simulink model "Integ_Model_Hepta"  (R2022a)
settings: configuration reference "VLS_Standard_Configuration" (kept outside this file)
undefined symbols (not defined in the file or in its folder): C_AFS_SpeedThrAct, C_AfsRampTimeMatrix, C_AnimationOnLoop, C_AnimationPeriod, C_AnimationPriority, C_CieCurveGammaToPwmY, C_CieCurvePwmToGammaY, C_CL_Ti_Speed_Hystresis, C_CL_Ti_Speed_Threshold, C_ClActAlgo, C_ClLeftSideTable_Alpha1, C_ClLeftSideTable_Alpha2, C_ClManeuverPwm, C_ClRightSideTable_Alpha1, C_ClRightSideTable_Alpha2, C_ClSpeedCurve, C_ClTableSize, C_ClTownPwm, C_Config, C_CSpeed0, C_DblDeadZone, C_DblEnable, C_DblInterDblAngValues, C_DblInterStwAngValues, C_DblLeftAngles, C_DblRampTime, C_DblRateLimit, C_DblRightAngles, C_DblSlavePeriod, C_DblSpeed0, C_DefaultValue, C_DrlRampTime, C_EndIndexOfEachLightingModule, C_EndValues, C_ForceExternalAfsMode, C_IndexOfStartStepForEachScenario, C_IsClOnTps, C_IsDblActive, C_IsDrlAutorizedInPower2, C_IsDrlPlOnTps, C_IsPlAutorizedInPower2, C_IsTiAutorizedInPower2, C_IsTiOnTps, C_LedCenterDist, C_LedCenterLimits, C_LedLeftDist, C_LedRightDist, C_LedStartIndexOfCl, C_LedStartIndexOfDrlPl, C_LedStartIndexOfTi, C_LeftDblMaxAngle, C_LeftDblMinAngle, C_MaintainAnimationPwm, C_MaintainAnimationTime, C_NumOfStepsForEachScenario, C_PlNominalPwm, C_PlOverDRL, C_RightDblMaxAngle, C_RightDblMinAngle, C_StartIndexOfEachLightingModule ... (+14)
libraries: simulink x11, AFS_MasterFeature x2, DodecaPreprocessingLib x1, Cl_Lib x1, DBL_MasterLib x1, AfsSlaveLib x1, DblSlaveLib x1, StdAnimationLibrary_R2020b x1, Ramp_Library_R2017b x1, STD_Signaling_Lib x1
(part 2 of 2)

== system Integ_Model_Hepta/Subsystem/Master/DBL_Master/Function-Call Subsystem ==
  V_FiltStWhAngleScaled : Inport
  V_DblEnable : Inport  Port=2
  V_FiltVehSpeed : Inport  Port=3
  function : TriggerPort  TriggerType=function-call  VariantControl=Variant
  Constant : Constant  Value=C_DblInterStwAngValues  VectorParams1D=off
  Constant1 : Constant  Value=C_DblDeadZone  VectorParams1D=off
  Constant2 : Constant  Value=C_DblInterDblAngValues  VectorParams1D=off
  Constant3 : Constant  Value=C_DblRateLimit  VectorParams1D=off
  Constant4 : Constant  Value=C_DblSpeed0  VectorParams1D=off
  Constant5 : Constant  Value=C_CSpeed0  VectorParams1D=off
  Constant6 : Constant  Value=C_LeftDblMinAngle  VectorParams1D=off
  Constant7 : Constant  Value=C_LeftDblMaxAngle  VectorParams1D=off
  Constant8 : Constant  Value=C_RightDblMinAngle  VectorParams1D=off
  Constant9 : Constant  Value=C_RightDblMaxAngle  VectorParams1D=off
  DblMasterLib : DBL_MasterLib/DblMasterLib  SystemSampleTime=-1  VariantActivationTime=update diagram  Latency=0  AutoFrameSizeCalculation=off
  V_LeftDblAimingAngle : Outport  VectorParamsAs1DForOutWhenUnconnected=off
  V_RightDblAimingAngle : Outport  Port=2  VectorParamsAs1DForOutWhenUnconnected=off
  wires:
  Constant7/1 -> DblMasterLib/11
  Constant4/1 -> DblMasterLib/8
  Constant6/1 -> DblMasterLib/10
  Constant9/1 -> DblMasterLib/13
  Constant5/1 -> DblMasterLib/9
  DblMasterLib/1 -> V_LeftDblAimingAngle/1
  V_DblEnable/1 -> DblMasterLib/2
  Constant2/1 -> DblMasterLib/4
  DblMasterLib/2 -> V_RightDblAimingAngle/1
  Constant1/1 -> DblMasterLib/5
  Constant/1 -> DblMasterLib/3
  V_FiltVehSpeed/1 -> DblMasterLib/7
  Constant3/1 -> DblMasterLib/6
  V_FiltStWhAngleScaled/1 -> DblMasterLib/1
  Constant8/1 -> DblMasterLib/12

== system Integ_Model_Hepta/Subsystem/SideDetection/SideDetectionManager/If Action Subsystem ==
  V_DblAimingAngleLeft : Inport
  V_CmdTiLeft : Inport  Port=2
  V_AfsMode : Inport  Port=3
  V_ClLeft : Inport  Port=4
  Action Port : ActionPort  ActionPortLabel=if(u1 == 0)
  V_DblAngle : Outport
  V_CmdTi : Outport  Port=2
  V_AfsLightingMode : Outport  Port=3
  V_ClActive : Outport  Port=4
  wires:
  V_DblAimingAngleLeft/1 -> V_DblAngle/1
  V_CmdTiLeft/1 -> V_CmdTi/1
  V_AfsMode/1 -> V_AfsLightingMode/1
  V_ClLeft/1 -> V_ClActive/1

== system Integ_Model_Hepta/Subsystem/SideDetection/SideDetectionManager/If Action Subsystem1 ==
  V_DblAimingAngleRight : Inport
  V_CmdTiRight : Inport  Port=2
  V_AfsModeCanIn : Inport  Port=3
  V_ClRight : Inport  Port=4
  Action Port : ActionPort  ActionPortLabel=else
  V_DblAngle : Outport
  V_CmdTi : Outport  Port=2
  V_AfsLightingMode : Outport  Port=3
  V_ClActive : Outport  Port=4
  wires:
  V_CmdTiRight/1 -> V_CmdTi/1
  V_DblAimingAngleRight/1 -> V_DblAngle/1
  V_AfsModeCanIn/1 -> V_AfsLightingMode/1
  V_ClRight/1 -> V_ClActive/1

== system Integ_Model_Hepta/Subsystem/Slave/AFS/ConvertAfsModetoSlave ==
  note: The requirement of different LB current
  V_ActiveLightingMode : Inport
  V_LowBeamRequest : Inport  Port=2
  Constant1 : Constant  Value=N_E_HBHighSpeed
  Constant12 : Constant  Value=N_E_HBLowSpeed
  Constant2 : Constant  Value=N_E_HBLowSpeed
  Constant21 : Constant  Value=0  OutDataTypeStr=Inherit: Inherit via back propagation
  Constant4 : Constant  Value=N_E_NoFunction
  Constant5 : Constant  Value=N_E_HBHighSpeed
  Constant6 : Constant  Value=0  OutDataTypeStr=Inherit: Inherit via back propagation
  Equal1 : RelationalOperator  Operator===  OutDataTypeStr=boolean  RndMeth=Simplest  InputSameDT=off
  Equal2 : RelationalOperator  Operator===  OutDataTypeStr=boolean  RndMeth=Simplest  InputSameDT=off
  Equal3 : RelationalOperator  Operator=~=  OutDataTypeStr=boolean  RndMeth=Simplest  InputSameDT=off
  Equal4 : RelationalOperator  Operator===  OutDataTypeStr=boolean  RndMeth=Simplest  InputSameDT=off
  Switch{,1..4} (5 alike) : Switch  Criteria=u2 ~= 0  SaturateOnIntegerOverflow=off  InputSameDT=off
  Vector Concatenate : Concatenate
  V_ActiveLightingModes : Outport
  wires:
  Switch/1 -> Vector Concatenate/2
  Constant12/1 -> Equal1/1, Switch3/1
  Constant21/1 -> Switch/1
  Vector Concatenate/1 -> V_ActiveLightingModes/1
  Equal2/1 -> Switch/2
  Switch1/1 -> Switch/3
  Equal3/1 -> Switch1/2
  Constant2/1 -> Switch2/1, Equal3/1
  V_ActiveLightingMode/1 -> Equal2/1, Equal3/2, Switch1/1, Equal1/2, Switch4/1, Equal4/1
  Switch2/1 -> Switch1/3
  V_LowBeamRequest/1 -> Switch2/2
  Constant4/1 -> Switch2/3
  Equal1/1 -> Switch3/2
  Switch3/1 -> Vector Concatenate/1
  Constant1/1 -> Equal2/2
  Switch4/1 -> Switch3/3
  Equal4/1 -> Switch4/2
  Constant5/1 -> Equal4/2
  Constant6/1 -> Switch4/3

== system Integ_Model_Hepta/Subsystem/Slave/Signaling/DrlPl ==
  Pl : Inport
  Drl : Inport  Port=2
  Constant : Constant  Value=C_PlNominalPwm
  Constant1 : Constant  Value=N_MaxPwm
  Constant2 : Constant  Value=0  OutDataTypeStr=Inherit: Inherit via back propagation
  Constant5 : Constant  Value=C_DrlRampTime
  Constant6 : Constant  Value=C_TeAdbSlave
  Constant7 : Constant  Value=C_CieCurvePwmToGammaY
  Constant8 : Constant  Value=C_CieCurveGammaToPwmY
  GammaRampLibraryPerLedGroup : Ramp_Library_R2017b/GammaRampLibraryPerLedGroup  Description=|  SystemSampleTime=-1  VariantActivationTime=update diagram  Latency=0  AutoFrameSizeCalculation=off
      | This library performs ramp function taking CIE curves which are evenly distributed.
      | It performs the ramp linearly on the Gamma Curve.
  Logical Operator : Logic  Operator=NOT  AllPortsSameDT=off  OutDataTypeStr=boolean
  Switch : Switch  Criteria=u2 ~= 0  OutDataTypeStr=Inherit: Inherit via back propagation  SaturateOnIntegerOverflow=off  InputSameDT=off
  Switch1 : Switch  Criteria=u2 ~= 0  OutDataTypeStr=Inherit: Inherit via back propagation  SaturateOnIntegerOverflow=off  InputSameDT=off
  Terminator : Terminator
  V_DrlPlTpsPwm : Outport
  wires:
  Switch/1 -> GammaRampLibraryPerLedGroup/1
  [Drl] -> Switch1/2
  Constant8/1 -> GammaRampLibraryPerLedGroup/6
  Constant1/1 -> Switch1/1
  Constant7/1 -> GammaRampLibraryPerLedGroup/5
  Drl/1 -> [Drl]
  Switch1/1 -> Switch/3
  Constant/1 -> Switch/1
  Constant5/1 -> GammaRampLibraryPerLedGroup/2
  [Drl] -> Logical Operator/1
  Constant6/1 -> GammaRampLibraryPerLedGroup/4
  Logical Operator/1 -> GammaRampLibraryPerLedGroup/3
  Constant2/1 -> Switch1/3
  Pl/1 -> Switch/2
  GammaRampLibraryPerLedGroup/2 -> Terminator/1
  GammaRampLibraryPerLedGroup/1 -> V_DrlPlTpsPwm/1

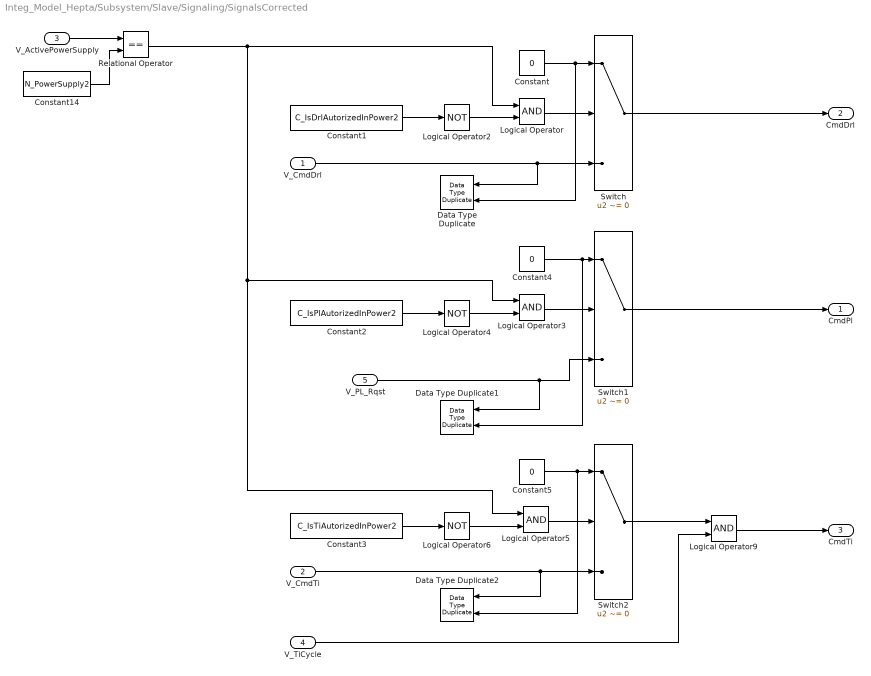
== system Integ_Model_Hepta/Subsystem/Slave/Signaling/SignalsCorrected ==
  "V_CmdDrl " : Inport
  V_CmdTi : Inport  Port=2
  V_ActivePowerSupply : Inport  Port=3
  V_TiCycle : Inport  Port=4
  V_PL_Rqst : Inport  Port=5
  Constant : Constant  Value=0  OutDataTypeStr=Inherit: Inherit via back propagation
  Constant1 : Constant  Value=C_IsDrlAutorizedInPower2
  Constant14 : Constant  Value=N_PowerSupply2
  Constant2 : Constant  Value=C_IsPlAutorizedInPower2
  Constant3 : Constant  Value=C_IsTiAutorizedInPower2
  Constant4 : Constant  Value=0  OutDataTypeStr=Inherit: Inherit via back propagation
  Constant5 : Constant  Value=0  OutDataTypeStr=Inherit: Inherit via back propagation
  Data Type Duplicate : DataTypeDuplicate
  Data Type Duplicate1 : DataTypeDuplicate
  Data Type Duplicate2 : DataTypeDuplicate
  Logical Operator{,3,5,9} (4 alike) : Logic  AllPortsSameDT=off  OutDataTypeStr=boolean
  Logical Operator2 : Logic  Operator=NOT  AllPortsSameDT=off  OutDataTypeStr=boolean
  Logical Operator4 : Logic  Operator=NOT  AllPortsSameDT=off  OutDataTypeStr=boolean
  Logical Operator6 : Logic  Operator=NOT  AllPortsSameDT=off  OutDataTypeStr=boolean
  Relational Operator : RelationalOperator  Operator===  OutDataTypeStr=boolean  RndMeth=Simplest  InputSameDT=off
  Switch : Switch  Criteria=u2 ~= 0  OutDataTypeStr=Inherit: Inherit via back propagation  SaturateOnIntegerOverflow=off  InputSameDT=off
  Switch1 : Switch  Criteria=u2 ~= 0  OutDataTypeStr=Inherit: Inherit via back propagation  SaturateOnIntegerOverflow=off  InputSameDT=off
  Switch2 : Switch  Criteria=u2 ~= 0  OutDataTypeStr=Inherit: Inherit via back propagation  SaturateOnIntegerOverflow=off  InputSameDT=off
  CmdPl : Outport
  CmdDrl : Outport  Port=2
  CmdTi : Outport  Port=3
  wires:
  Constant3/1 -> Logical Operator6/1
  V_TiCycle/1 -> Logical Operator9/2
  Switch1/1 -> CmdPl/1
  Switch2/1 -> Logical Operator9/1
  Logical Operator6/1 -> Logical Operator5/2
  Switch/1 -> CmdDrl/1
  Logical Operator9/1 -> CmdTi/1
  Logical Operator4/1 -> Logical Operator3/2
  V_ActivePowerSupply/1 -> Relational Operator/1
  Logical Operator3/1 -> Switch1/2
  Constant14/1 -> Relational Operator/2
  Relational Operator/1 -> Logical Operator5/1, Logical Operator3/1, Logical Operator/1
  Constant1/1 -> Logical Operator2/1
  "V_CmdDrl "/1 -> Data Type Duplicate/1, Switch/3
  Constant4/1 -> Data Type Duplicate1/2, Switch1/1
  Constant5/1 -> Data Type Duplicate2/2, Switch2/1
  V_PL_Rqst/1 -> Data Type Duplicate1/1, Switch1/3
  Logical Operator5/1 -> Switch2/2
  Logical Operator/1 -> Switch/2
  Logical Operator2/1 -> Logical Operator/2
  V_CmdTi/1 -> Data Type Duplicate2/1, Switch2/3
  Constant2/1 -> Logical Operator4/1
  Constant/1 -> Data Type Duplicate/2, Switch/1

== system Integ_Model_Hepta/Subsystem/Slave/Signaling/Ti ==
  Ti : Inport
  Constant3 : Constant  Value=N_MaxPwm
  Constant4 : Constant  Value=0  OutDataTypeStr=Inherit: Inherit via back propagation
  Switch2 : Switch  Criteria=u2 ~= 0  OutDataTypeStr=Inherit: Inherit via back propagation  SaturateOnIntegerOverflow=off  InputSameDT=off
  V_TiTpsPwm : Outport
  wires:
  Constant4/1 -> Switch2/3
  Constant3/1 -> Switch2/1
  Ti/1 -> Switch2/2
  Switch2/1 -> V_TiTpsPwm/1

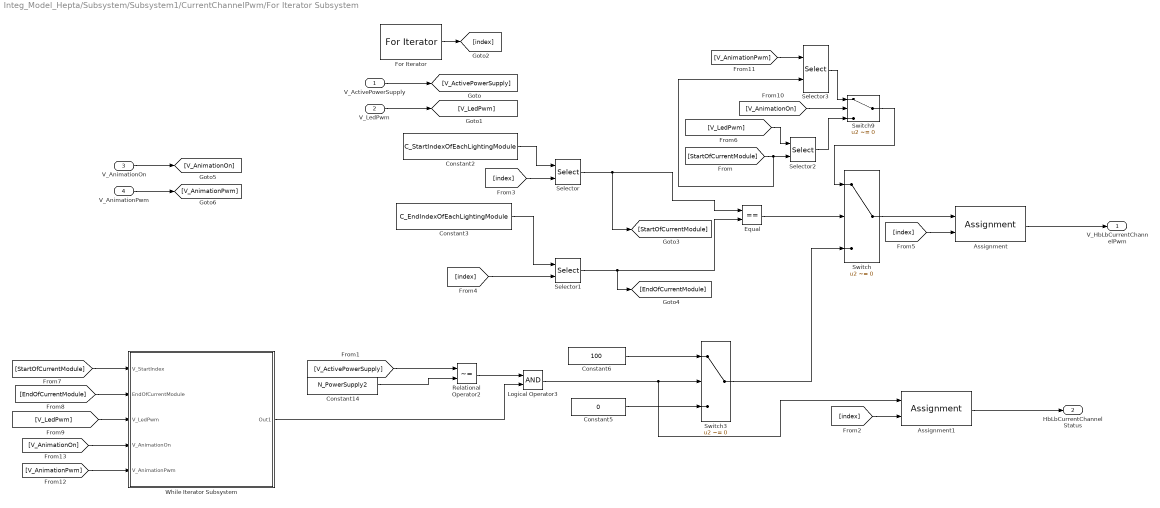
== system Integ_Model_Hepta/Subsystem/Subsystem1/CurrentChannelPwm/For Iterator Subsystem ==
  V_ActivePowerSupply : Inport
  V_LedPwm : Inport  Port=2
  V_AnimationOn : Inport  Port=3
  V_AnimationPwm : Inport  Port=4
  Assignment : Assignment  IndexMode=Zero-based  OutputInitialize=Specify size for each dimension in table  DiagnosticForDimensions=Error  IndexOptions=Starting index (port)  Indices=1  OutputSizes=C_NumOfLightingModules
  Assignment1 : Assignment  IndexMode=Zero-based  OutputInitialize=Specify size for each dimension in table  DiagnosticForDimensions=Error  IndexOptions=Starting index (port)  Indices=1  OutputSizes=C_NumOfLightingModules
  Constant14 : Constant  Value=N_PowerSupply2  OutDataTypeStr=Inherit: Inherit via back propagation
  Constant2 : Constant  Value=C_StartIndexOfEachLightingModule
  Constant3 : Constant  Value=C_EndIndexOfEachLightingModule
  Constant5 : Constant  Value=0
  Constant6 : Constant  Value=100  OutDataTypeStr=Inherit: Inherit via back propagation
  Equal : RelationalOperator  Operator===  OutDataTypeStr=boolean  RndMeth=Simplest  InputSameDT=off
  For Iterator : ForIterator  IterationLimit=C_NumOfLightingModules  IndexMode=Zero-based
  Logical Operator3 : Logic  AllPortsSameDT=off  OutDataTypeStr=boolean
  Relational Operator2 : RelationalOperator  Operator=~=  OutDataTypeStr=boolean  RndMeth=Simplest  InputSameDT=off
  Selector{,1..3} (4 alike) : Selector  IndexMode=Zero-based  IndexOptions=Index vector (port)  Indices=[1 3]  OutputSizes=1
  Switch : Switch  Criteria=u2 ~= 0  SaturateOnIntegerOverflow=off  InputSameDT=off
  Switch3 : Switch  Criteria=u2 ~= 0  SaturateOnIntegerOverflow=off  InputSameDT=off
  Switch9 : Switch  Criteria=u2 ~= 0  SaturateOnIntegerOverflow=off  InputSameDT=off
  While Iterator Subsystem : Subsystem  TreatAsAtomicUnit=on
  V_HbLbCurrentChannelPwm : Outport
  HbLbCurrentChannelStatus : Outport  Port=2
  wires:
  Selector/1 -> [StartOfCurrentModule], Equal/1
  Selector1/1 -> [EndOfCurrentModule], Equal/2
  Equal/1 -> Switch/2
  V_ActivePowerSupply/1 -> [V_ActivePowerSupply]
  V_LedPwm/1 -> [V_LedPwm]
  Selector2/1 -> Switch9/3
  Constant14/1 -> Relational Operator2/2
  Constant6/1 -> Switch3/1
  Switch3/1 -> Switch/3
  Relational Operator2/1 -> Logical Operator3/1
  Constant5/1 -> Switch3/3
  Logical Operator3/1 -> Assignment1/1, Switch3/2
  While Iterator Subsystem/1(Out1) -> Logical Operator3/2
  [V_ActivePowerSupply] -> Relational Operator2/1
  Switch/1 -> Assignment/1
  For Iterator/1 -> [index]
  [index] -> Selector/2
  [index] -> Selector1/2
  Constant2/1 -> Selector/1
  Constant3/1 -> Selector1/1
  Assignment/1 -> V_HbLbCurrentChannelPwm/1
  [index] -> Assignment/2
  [V_LedPwm] -> Selector2/1
  [StartOfCurrentModule] -> Selector3/2, Selector2/2
  [StartOfCurrentModule] -> While Iterator Subsystem/1(V_StartIndex)
  [EndOfCurrentModule] -> While Iterator Subsystem/2(EndOfCurrentModule)
  [V_LedPwm] -> While Iterator Subsystem/3(V_LedPwm)
  [index] -> Assignment1/2
  Assignment1/1 -> HbLbCurrentChannelStatus/1
  Selector3/1 -> Switch9/1
  V_AnimationPwm/1 -> [V_AnimationPwm]
  V_AnimationOn/1 -> [V_AnimationOn]
  [V_AnimationOn] -> Switch9/2
  [V_AnimationPwm] -> Selector3/1
  Switch9/1 -> Switch/1
  [V_AnimationPwm] -> While Iterator Subsystem/5(V_AnimationPwm)
  [V_AnimationOn] -> While Iterator Subsystem/4(V_AnimationOn)

== system Integ_Model_Hepta/Subsystem/Subsystem1/CurrentChannelPwm/Subsystem2 ==
  V_DrlPlFunctionTpsPwm : Inport
  V_PL_OUT : Inport  Port=2
  V_DRL_OUT : Inport  Port=3
  V_AnimationOn : Inport  Port=4
  If : If  NumInputs=2  IfExpression=u1==1  ElseIfExpressions=u2==1
  If Action Subsystem : Subsystem  TreatAsAtomicUnit=on
  If Action Subsystem1 : Subsystem  TreatAsAtomicUnit=on
  If Action Subsystem2 : Subsystem  TreatAsAtomicUnit=on
  IsNonZero : simulink/Logic and Bit Operations/Compare To Zero  relop=~=  OutDataTypeStr=boolean
  IsNonZero1 : simulink/Logic and Bit Operations/Compare To Zero  relop=~=  OutDataTypeStr=boolean
  Logical Operator : Logic  AllPortsSameDT=off  OutDataTypeStr=boolean
  Logical Operator1 : Logic  AllPortsSameDT=off  OutDataTypeStr=boolean
  Logical Operator2 : Logic  Operator=OR  AllPortsSameDT=off  OutDataTypeStr=boolean
  Merge : Merge  Inputs=3
  Channle_Status : Outport
  wires:
  V_PL_OUT/1 -> Logical Operator/2
  If/1 -> If Action Subsystem/Action
  Merge/1 -> Channle_Status/1
  V_DrlPlFunctionTpsPwm/1 -> Logical Operator/1, Logical Operator1/2
  If/2 -> If Action Subsystem1/Action
  Logical Operator1/1 -> IsNonZero1/1
  IsNonZero/1 -> If/2
  If/3 -> If Action Subsystem2/Action
  V_DRL_OUT/1 -> Logical Operator2/2
  If Action Subsystem2/1(Channle_Status) -> Merge/3
  Logical Operator/1 -> IsNonZero/1
  If Action Subsystem/1(Channle_Status) -> Merge/1
  IsNonZero1/1 -> If/1
  If Action Subsystem1/1(Channle_Status) -> Merge/2
  Logical Operator2/1 -> Logical Operator1/1
  V_AnimationOn/1 -> Logical Operator2/1

== system Integ_Model_Hepta/Subsystem/Master/AFS_Master/AFS_Master/AFS_Fail_safe_strategy ==
  V_CAN_Fail : Inport
  V_Veh_speed_Fail : Inport  Port=2
  V_Mod_LeftFail : Inport  Port=3
  V_Mod_RightFail : Inport  Port=4
  V_AFS_ActStatus : Inport  Port=5
  V_FiltVehSpeed : Inport  Port=6
  function : TriggerPort  TriggerType=function-call  VariantControl=Variant
  AFS_Fail_safe_strategy : Subsystem  Description=AFS_Fail_safe_strategy
  V_AFS_OperatState : Outport  VectorParamsAs1DForOutWhenUnconnected=off
  V_AFS_Fail : Outport  Port=2  VectorParamsAs1DForOutWhenUnconnected=off
  wires:
  V_FiltVehSpeed/1 -> AFS_Fail_safe_strategy/6(V_FiltVehSpeed)
  AFS_Fail_safe_strategy/1(V_AFS_OperatState) -> V_AFS_OperatState/1
  AFS_Fail_safe_strategy/2(V_AFS_Fail) -> V_AFS_Fail/1
  V_Mod_RightFail/1 -> AFS_Fail_safe_strategy/4(V_Mod_RightFail)
  V_Mod_LeftFail/1 -> AFS_Fail_safe_strategy/3(V_Mod_LeftFail)
  V_AFS_ActStatus/1 -> AFS_Fail_safe_strategy/5(V_AFS_ActStatus)
  V_CAN_Fail/1 -> AFS_Fail_safe_strategy/1(V_CAN_Fail)
  V_Veh_speed_Fail/1 -> AFS_Fail_safe_strategy/2(V_Veh_speed_Fail)

== system Integ_Model_Hepta/Subsystem/Master/AFS_Master/AFS_Master/AfsModeManager ==
  ForceExternalAfsMode : Inport
  ExternalAfsMode : Inport  Port=2
  V_LbStatus : Inport  Port=3
  V_AFS_OperatState : Inport  Port=4
  V_ActivateADBFeatures : Inport  Port=5
  V_FiltVehSpeed : Inport  Port=6
  V_WetDetection : Inport  Port=7
  V_TouristModeActivated : Inport  Port=8
  V_Foggy : Inport  Port=9
  V_RevGearEng : Inport  Port=10
  V_DayNightStatus : Inport  Port=11
  V_HBNoADBRequest : Inport  Port=12
  function : TriggerPort  TriggerType=function-call  VariantControl=Variant
  AFS_Manager : AFS_MasterFeature/AFS_Manager  Description=AFS_Subsystem  SystemSampleTime=-1  VariantActivationTime=update diagram  Latency=0  AutoFrameSizeCalculation=off
  V_AfsMode : Outport  PortDimensions=1
  wires:
  V_HBNoADBRequest/1 -> AFS_Manager/12
  V_DayNightStatus/1 -> AFS_Manager/11
  V_AFS_OperatState/1 -> AFS_Manager/4
  V_RevGearEng/1 -> AFS_Manager/10
  AFS_Manager/1 -> V_AfsMode/1
  V_Foggy/1 -> AFS_Manager/9
  V_TouristModeActivated/1 -> AFS_Manager/8
  V_WetDetection/1 -> AFS_Manager/7
  V_FiltVehSpeed/1 -> AFS_Manager/6
  V_ActivateADBFeatures/1 -> AFS_Manager/5
  V_LbStatus/1 -> AFS_Manager/3
  ForceExternalAfsMode/1 -> AFS_Manager/1
  ExternalAfsMode/1 -> AFS_Manager/2

== system Integ_Model_Hepta/Subsystem/Master/Cl_Master/CL_MasterFunction/Cl_Master_func_Call ==
  V_TiLeft : Inport
  V_TiRight : Inport  Port=2
  V_FiltVehSpeed : Inport  Port=3
  V_CurveRadius : Inport  Port=4
  V_FiltStWhAngleScaled : Inport  Port=5
  ClActivation1 : Cl_Lib/ClActivation  SystemSampleTime=-1  VariantActivationTime=update diagram  Latency=0  AutoFrameSizeCalculation=off
  Constant : Constant  OutDataTypeStr=Inherit: Inherit via back propagation
  Constant1 : Constant  Value=C_CL_Ti_Speed_Hystresis
  Constant10 : Constant  Value=C_ClSpeedCurve
  Constant11 : Constant  Value=C_CL_Ti_Speed_Threshold
  Constant12 : Constant  Value=C_ClLeftSideTable_Alpha2
  Constant13 : Constant  Value=C_ClActAlgo
  Constant3 : Constant  Value=C_ClTableSize
  Constant5 : Constant  Value=C_ClLeftSideTable_Alpha1
  Constant6 : Constant  Value=C_ClRightSideTable_Alpha2
  Constant7 : Constant  Value=C_TickTIBlk
  Constant8 : Constant  Value=C_ClRightSideTable_Alpha1
  V_ClRight : Outport
  V_ClLeft : Outport  Port=2
  wires:
  V_TiRight/1 -> ClActivation1/2
  V_FiltVehSpeed/1 -> ClActivation1/3
  ClActivation1/1 -> V_ClRight/1
  V_CurveRadius/1 -> ClActivation1/4
  V_TiLeft/1 -> ClActivation1/1
  V_FiltStWhAngleScaled/1 -> ClActivation1/5
  ClActivation1/2 -> V_ClLeft/1
  Constant7/1 -> ClActivation1/7
  Constant11/1 -> ClActivation1/8
  Constant1/1 -> ClActivation1/9
  Constant10/1 -> ClActivation1/10
  Constant8/1 -> ClActivation1/11
  Constant5/1 -> ClActivation1/12
  Constant6/1 -> ClActivation1/13
  Constant12/1 -> ClActivation1/14
  Constant3/1 -> ClActivation1/15
  Constant13/1 -> ClActivation1/16
  Constant/1 -> ClActivation1/6

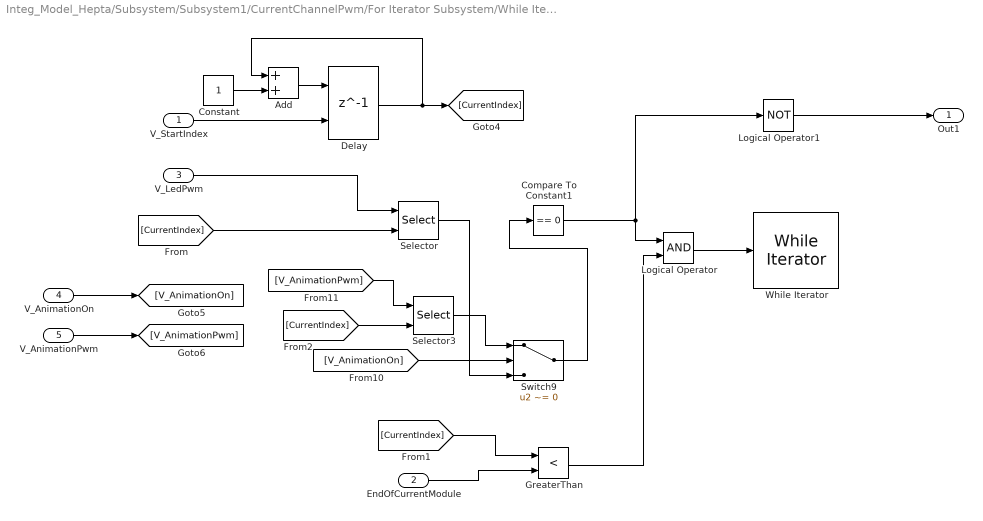
== system Integ_Model_Hepta/Subsystem/Subsystem1/CurrentChannelPwm/For Iterator Subsystem/While Iterator Subsystem ==
  V_StartIndex : Inport
  EndOfCurrentModule : Inport  Port=2
  V_LedPwm : Inport  Port=3
  V_AnimationOn : Inport  Port=4
  V_AnimationPwm : Inport  Port=5
  Add : Sum  AccumDataTypeStr=uint32  OutDataTypeStr=uint32
  Compare To Constant1 : simulink/Logic and Bit Operations/Compare To Constant  relop===  const=0  OutDataTypeStr=boolean
  Constant : Constant  OutDataTypeStr=uint8
  Delay : Delay  DelayLength=1  InitialConditionSource=Input port
      settings: InputPortMap=u0,p4
  GreaterThan : RelationalOperator  Operator=<  OutDataTypeStr=boolean  RndMeth=Simplest  InputSameDT=off
  Logical Operator : Logic  AllPortsSameDT=off  OutDataTypeStr=boolean
  Logical Operator1 : Logic  Operator=NOT  AllPortsSameDT=off  OutDataTypeStr=boolean
  Selector : Selector  IndexMode=Zero-based  IndexOptions=Index vector (port)  Indices=[1 3]  OutputSizes=1
  Selector3 : Selector  IndexMode=Zero-based  IndexOptions=Index vector (port)  Indices=[1 3]  OutputSizes=1
  Switch9 : Switch  Criteria=u2 ~= 0  SaturateOnIntegerOverflow=off  InputSameDT=off
  While Iterator : WhileIterator  MaxIters=-1  WhileBlockType=do-while  ResetStates=reset
  Out1 : Outport
  wires:
  Compare To Constant1/1 -> Logical Operator/1, Logical Operator1/1
  V_StartIndex/1 -> Delay/2
  Add/1 -> Delay/1
  Delay/1 -> [CurrentIndex], Add/1
  Constant/1 -> Add/2
  [CurrentIndex] -> Selector/2
  V_LedPwm/1 -> Selector/1
  Switch9/1 -> Compare To Constant1/1
  [CurrentIndex] -> GreaterThan/1
  EndOfCurrentModule/1 -> GreaterThan/2
  GreaterThan/1 -> Logical Operator/2
  Logical Operator/1 -> While Iterator/1
  Logical Operator1/1 -> Out1/1
  V_AnimationPwm/1 -> [V_AnimationPwm]
  V_AnimationOn/1 -> [V_AnimationOn]
  [V_AnimationPwm] -> Selector3/1
  [CurrentIndex] -> Selector3/2
  [V_AnimationOn] -> Switch9/2
  Selector3/1 -> Switch9/1
  Selector/1 -> Switch9/3

== system Integ_Model_Hepta/Subsystem/Subsystem1/CurrentChannelPwm/Subsystem2/If Action Subsystem ==
  Action Port : ActionPort  ActionPortLabel=if(u1==1)
  Constant2 : Constant  OutDataTypeStr=uint8
  Channle_Status : Outport
  wires:
  Constant2/1 -> Channle_Status/1

== system Integ_Model_Hepta/Subsystem/Subsystem1/CurrentChannelPwm/Subsystem2/If Action Subsystem1 ==
  Action Port : ActionPort  ActionPortLabel=elseif(u2==1)
  Constant2 : Constant  OutDataTypeStr=uint8
  Channle_Status : Outport
  wires:
  Constant2/1 -> Channle_Status/1

== system Integ_Model_Hepta/Subsystem/Subsystem1/CurrentChannelPwm/Subsystem2/If Action Subsystem2 ==
  Action Port : ActionPort  ActionPortLabel=else
  Constant2 : Constant  Value=0  OutDataTypeStr=uint8
  Channle_Status : Outport
  wires:
  Constant2/1 -> Channle_Status/1

== system Integ_Model_Hepta/Subsystem/Master/AFS_Master/AFS_Master/AFS_Fail_safe_strategy/AFS_Fail_safe_strategy ==
  V_CAN_Fail : Inport
  V_Veh_speed_Fail : Inport  Port=2
  V_Mod_LeftFail : Inport  Port=3
  V_Mod_RightFail : Inport  Port=4
  V_AFS_ActStatus : Inport  Port=5
  V_FiltVehSpeed : Inport  Port=6
  AFS_Fail_safe_strategy : AFS_MasterFeature/AFS_Fail_safe_strategy  SystemSampleTime=-1  VariantActivationTime=update diagram  Latency=0  AutoFrameSizeCalculation=off
  Constant70 : Constant  Value=C_AFS_SpeedThrAct
  Logical Operator : Logic  Operator=OR  Inputs=4  AllPortsSameDT=off  OutDataTypeStr=boolean
  Relational Operator : RelationalOperator  OutDataTypeStr=boolean  RndMeth=Floor  InputSameDT=off
  V_AFS_OperatState : Outport  VectorParamsAs1DForOutWhenUnconnected=off
  V_AFS_Fail : Outport  Port=2  VectorParamsAs1DForOutWhenUnconnected=off
  wires:
  AFS_Fail_safe_strategy/1 -> V_AFS_OperatState/1
  Relational Operator/1 -> AFS_Fail_safe_strategy/3
  AFS_Fail_safe_strategy/2 -> V_AFS_Fail/1
  Constant70/1 -> Relational Operator/2
  Logical Operator/1 -> AFS_Fail_safe_strategy/1
  V_FiltVehSpeed/1 -> Relational Operator/1
  V_Mod_LeftFail/1 -> Logical Operator/3
  V_Veh_speed_Fail/1 -> Logical Operator/2
  V_CAN_Fail/1 -> Logical Operator/1
  V_AFS_ActStatus/1 -> AFS_Fail_safe_strategy/2
  V_Mod_RightFail/1 -> Logical Operator/4
